simulink model "pv_design"  (R2015a)
settings: Solver=ode45  StartTime=0.0  StopTime=10  RelTol=1e-3
libraries: powerlib x10, fuzblock x1, powerlib_meascontrol x1, re_lib x1
settings Model: Creator=Shanto  LastModifiedBy=Shanto

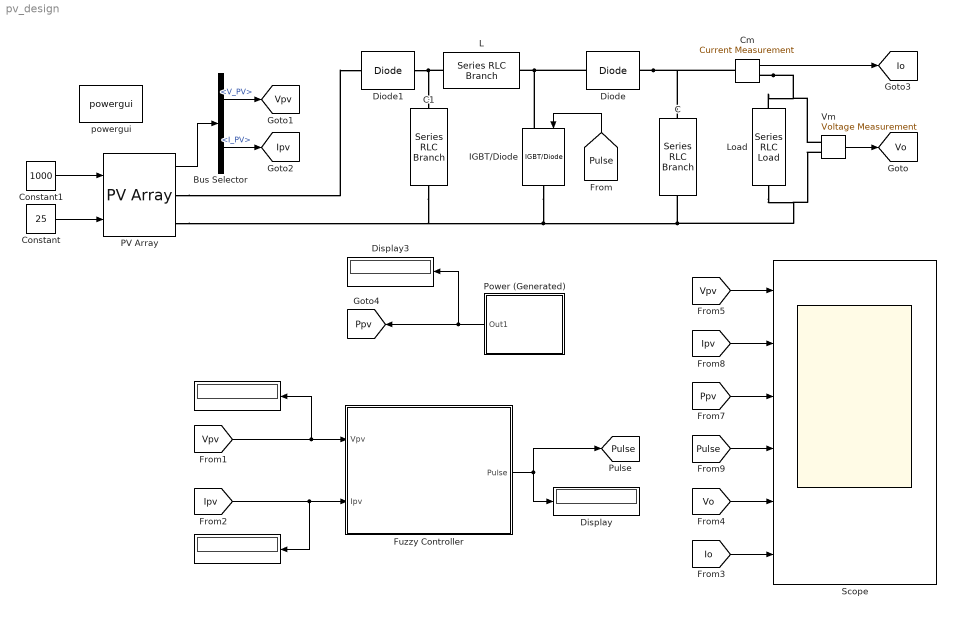
== system pv_design ==
  " " : Display
  "   " : Display
  " Load" : powerlib/Elements/Series RLC Load  LConnTagsString=a  RConnTagsString=__new0  NominalVoltage=30  NominalFrequency=50  ActivePower=120  InductivePower=0  CapacitivePower=0  Setx0=off  InitialVoltage=0  SetiL0=off  InitialCurrent=0  Measurements=None
  Bus Selector : BusSelector  OutputSignals=V_PV,I_PV
  C : powerlib/Elements/Series RLC Branch  LConnTagsString=__new0  RConnTagsString=__new0  BranchType=C  Resistance=1  Inductance=1e-3  SetiL0=off  InitialCurrent=0  Capacitance=50e-6  Setx0=off  InitialVoltage=0  Measurements=None
  C1 : powerlib/Elements/Series RLC Branch  LConnTagsString=__new0  RConnTagsString=__new0  BranchType=C  Resistance=1  Inductance=1e-3  SetiL0=off  InitialCurrent=0  Capacitance=4000e-6  Setx0=off  InitialVoltage=0  Measurements=None
  Cm : powerlib/Measurements/Current Measurement  PhasorSimulation=off  OutputType=Complex  PSBequivalent=0
  Constant : Constant  Value=25
  Constant1 : Constant  Value=1000
  Diode : powerlib/Power Electronics/Diode  Ron=0.001  Lon=0  Vf=0.8  IC=0  UseSnubber=off  Rs=500  Cs=250e-9  Measurements=off
  Diode1 : powerlib/Power Electronics/Diode  Ron=0.001  Lon=0  Vf=0.8  IC=0  UseSnubber=off  Rs=500  Cs=250e-9  Measurements=off
  Display : Display
  Display3 : Display
  Fuzzy Controller : Subsystem
  IGBT/Diode : powerlib/Power Electronics/IGBT//Diode  Ron=1e-3  Rs=1e5  Cs=inf  Measurements=off
  L : powerlib/Elements/Series RLC Branch  LConnTagsString=__new0  RConnTagsString=__new0  BranchType=L  Resistance=1  Inductance=1e-4  SetiL0=off  InitialCurrent=0  Capacitance=1e-6  Setx0=off  InitialVoltage=0  Measurements=None
  PV Array : re_lib/Solar/PV Array  Npar=1  Nser=1  PlotType=one module @ 25 deg.C & specified irradiances  S_vec="[ 1000  500  100 ]"  Temp_C_vec="[ 45 25  ]"  ModuleName=1Soltech 1STH-215-P  PlotWhenSelected=off  Pm=213.15  Ncell=60  Voc=36.3  Isc=7.84  Vm=29  Im=7.35  beta_Voc_pc=-0.36099  alpha_Isc_pc=0.102  beta_Voc=-0.13104  alpha_Isc=0.007997  IL=7.8649  I0=2.9259e-10  nI=0.98117  Rsh=313.3991  Rs=0.39383  BAL=on  Tc=1e-6  Tfilter=5e-5
  Power (Generated) : Subsystem
  Scope : Scope  NumInputPorts=6
      settings: YMin=8.5~7.824~65~0~10~1  YMax=9.5~7.828~75~1~30~4
  "Vm " : powerlib/Measurements/Voltage Measurement  PhasorSimulation=off  OutputType=Complex  PSBequivalent=0
  powergui : powerlib/powergui  Priority=1  SimulationMode=Discrete  SolverType=Tustin/Backward Euler (TBE)  SampleTime=50e-6  frequency=60  SPID=off  DisableSnubberDevices=off  DisableRonSwitches=off  DisableVfSwitches=off  SwTol=0  DisplayEquations=off  Interpol=off  methode=off  Ts=100  FunctionMessages=off  echomessages=off  HookPort=off  EnableUseOfTLC=off  x0status=blocks  frequencyindice=0  Pbase=100e6  ErrMax=1e-4  Iterations=50  UnitsV=kV  UnitsW=MW  buscounter=0  RestoreLinks=warning  ResistiveCurrentMeasurement=off  Frange=[0:2:500]  Ylog=off  Xlog=on  ShowGrid=off  save=off  variable=ZData  structure=0  ZoomFFT=off  StartTime=0.0  cycles=1  DisplayStyle=1  fundamental=60  FreqAxis=off  MaxFrequency=1000  frequencyindicesteady=1  RmsSteady=1  display=off
  tag scope: Io=global, Ipv=global, Ppv=global, Pulse=global, Vo=global, Vpv=global
  wires:
  Constant1/1 -> PV Array/1
  Constant/1 -> PV Array/2
  PV Array/1 -> Bus Selector/1
  Bus Selector/1 -> [Vpv]  "<V_PV>"
  Bus Selector/2 -> [Ipv]  "<I_PV>"
  [Pulse] -> IGBT/Diode/1
  [Ipv] -> " "/1, Fuzzy Controller/2(Ipv)
  [Vpv] -> "   "/1, Fuzzy Controller/1(Vpv)
  Fuzzy Controller/1(Pulse) -> [Pulse], Display/1
  Power (Generated)/1(Out1) -> [Ppv], Display3/1
  Cm/1 -> [Io]
  "Vm "/1 -> [Vo]
  [Ppv] -> Scope/3
  [Vpv] -> Scope/1
  [Ipv] -> Scope/2
  [Vo] -> Scope/5
  [Io] -> Scope/6
  [Pulse] -> Scope/4
  connections:
  Cm/RConn1 -- "Vm "/LConn1 -- " Load"/LConn1
  IGBT/Diode/RConn1 -- PV Array/RConn2 -- C1/RConn1 -- "Vm "/LConn2 -- " Load"/RConn1 -- C/RConn1
  L/LConn1 -- Diode/LConn1 -- IGBT/Diode/LConn1
  Diode1/RConn1 -- C1/LConn1 -- L/RConn1
  Diode/RConn1 -- Cm/LConn1 -- C/LConn1
  PV Array/RConn1 -- Diode1/LConn1

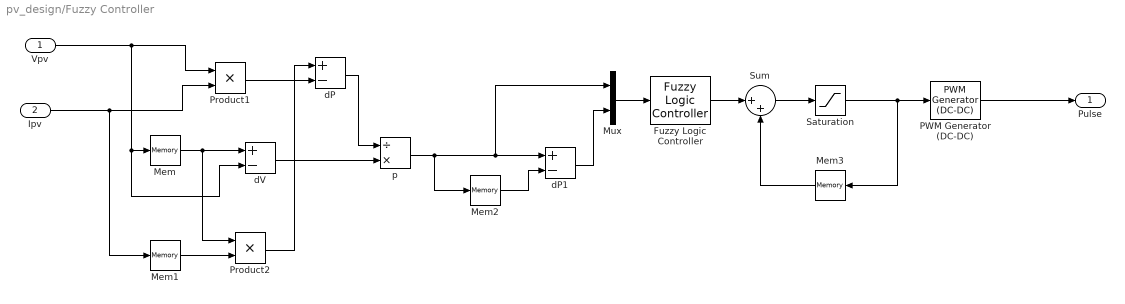
== system pv_design/Fuzzy Controller ==
  Vpv : Inport
  Ipv : Inport  Port=2
  Fuzzy Logic Controller : fuzblock/Fuzzy Logic  Controller  fis='po_mppt.fis'
  Mem{,1..3} (4 alike) : Memory
  Mux : Mux  Inputs=2
  PWM Generator (DC-DC) : powerlib_meascontrol/Pulse & Signal Generators/PWM Generator (DC-DC)  Fsw=5000  Ts=0
  Product1 : Product
  Product2 : Product
  Saturation : Saturate
  Sum : Sum  Inputs=|++
  dP : Sum  Inputs=+-
  dP1 : Sum  Inputs=+-
  dV : Sum  Inputs=+-
  p : Product  Inputs=/*
  Pulse : Outport
  wires:
  Ipv/1 -> Mem1/1, Product1/2
  Vpv/1 -> Mem/1, dV/2, Product1/1
  Sum/1 -> Saturation/1
  dP/1 -> p/1
  p/1 -> dP1/1, Mux/1, Mem2/1
  dP1/1 -> Mux/2
  Mem1/1 -> Product2/2
  Mux/1 -> Fuzzy Logic Controller/1
  Mem/1 -> dV/1, Product2/1
  Saturation/1 -> PWM Generator (DC-DC)/1, Mem3/1
  Product1/1 -> dP/2
  dV/1 -> p/2
  Fuzzy Logic Controller/1 -> Sum/1
  PWM Generator (DC-DC)/1 -> Pulse/1
  Mem2/1 -> dP1/2
  Mem3/1 -> Sum/2
  Product2/1 -> dP/1

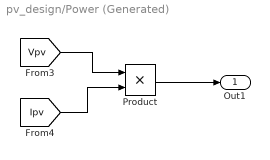
== system pv_design/Power (Generated) ==
  Product : Product
  Out1 : Outport
  wires:
  [Ipv] -> Product/2
  [Vpv] -> Product/1
  Product/1 -> Out1/1
